simulink library "Swerve_Modules_Controls_Lib"  (R2023a)
settings: Solver=VariableStepAuto  StartTime=0.0  StopTime=10.0  RelTol=1e-3
libraries: Swerve_Drive_lib x4, simulink_extras x4, Rotation2D x4, $bdroot x4, eeGeneralControl x1, slpidlib x1
settings Model: Creator=ander  LastModifiedBy=ander

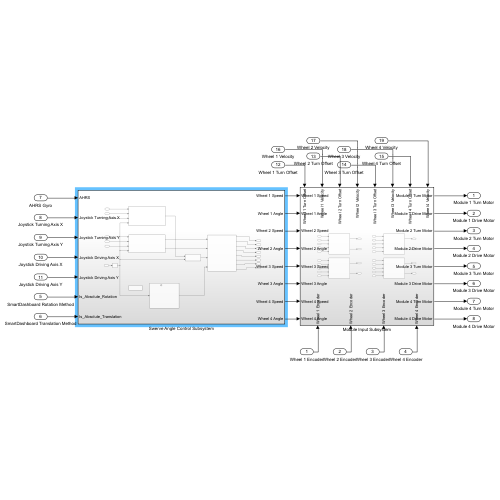
[thumbnail: Simulink's stored preview of the top-level diagram]
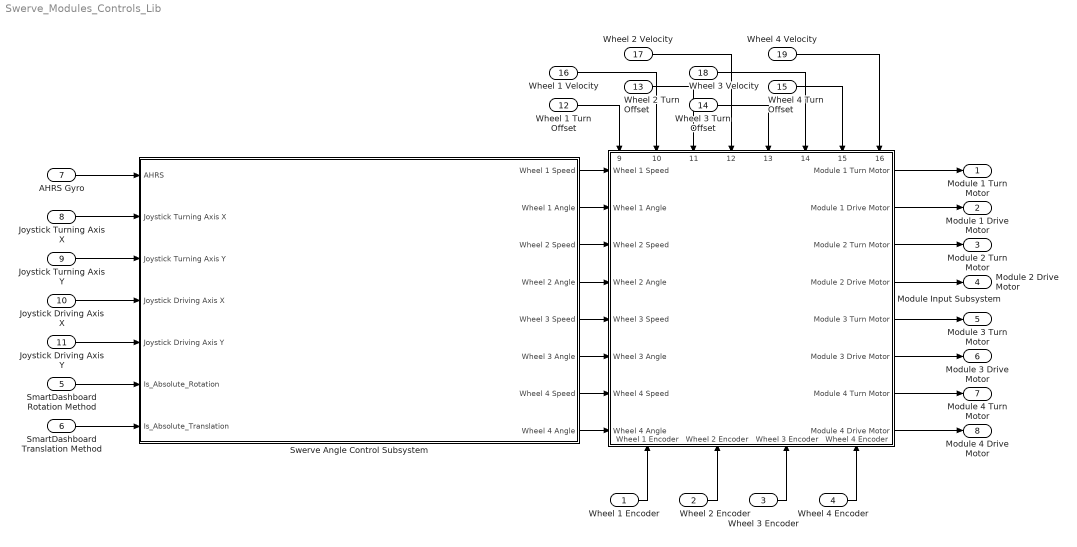
== system Swerve_Modules_Controls_Lib ==
  Wheel 1 Encoder : Inport
  Wheel 2 Encoder : Inport  Port=2
  Wheel 3 Encoder : Inport  Port=3
  Wheel 4 Encoder : Inport  Port=4
  SmartDashboard Rotation Method : Inport  Port=5
  SmartDashboard Translation Method : Inport  Port=6
  AHRS Gyro : Inport  Port=7
  Joystick Turning Axis X : Inport  Port=8
  Joystick Turning Axis Y : Inport  Port=9
  Joystick Driving Axis X : Inport  Port=10
  Joystick Driving Axis Y : Inport  Port=11
  Wheel 1 Turn Offset : Inport  Port=12
  Wheel 2 Turn Offset : Inport  Port=13
  Wheel 3 Turn Offset : Inport  Port=14
  Wheel 4 Turn Offset : Inport  Port=15
  Wheel 1 Velocity : Inport  Port=16
  Wheel 2 Velocity : Inport  Port=17
  Wheel 3 Velocity : Inport  Port=18
  Wheel 4 Velocity : Inport  Port=19
  Module Input Subsystem : Subsystem
      settings: PortSchema="{\"entries\":[{\"content\":{\"sides\":[{\"content\":{\"connectorIds\":[\"In1\",\"In2\",\"In3\",\"In4\",\"In5\",\"In6\",\"In7\",\"In8\"]},\"type\":\"ConnectorPlacement.EquallySpacedRectSide\",\"uuid\":\"43d98aa7-b040-4852-b29d-defb04b38bb2\"},{\"content\":{\"connectorIds\":[\"Out1\",\"Out2\",\"Out3\",\"Out4\",\"Out5\",\"Out6\",\"Out7\",\"Out8\"],\"side\":\"RIGHT\"},\"type\":\"ConnectorPlacement.EquallySpacedRectSide\",\"uuid\":\"cb41fb5c-ab8a-47da-953a-19fc3d1ad3d6\"},{\"content\":{\"connectorIds\":[\"In9\",\"In10\",\"In11\",\"In12\",\"In13\",\"In14\",\"In15\",\"In16\"],\"side\":\"TOP\"},\"type\":\"ConnectorPlacement.EquallySpacedRectSide\",\"uuid\":\"495c5582-c95d-45e8-a83d-3ddc2229b4de\"},{\"content\":{\"connectorIds\":[\"In17\",\"In18\",\"In19\",\"In20\"],\"side\":\"BOTTOM\"},\"type\":\"ConnectorPlacement.EquallySpacedRectSide\",\"uuid\":\"c356cfa6-29bf-4b1b-9842-1083247295af\"}]},\"type\":\"ConnectorPlacement.EquallySpacedConnector\",\"uuid\":\"1f745937-a7fb-445d-9d3d-b08fd0374c25\"}],\"packageUris\":[\"http://schema.mathworks.com/mf0/Connector/R2020b\"],\"version\":\"1.0\"}"
  Swerve Angle Control Subsystem : Subsystem
  Module 1 Turn Motor : Outport
  Module 1 Drive Motor : Outport  Port=2
  Module 2 Turn Motor : Outport  Port=3
  Module 2 Drive Motor : Outport  Port=4
  Module 3 Turn Motor : Outport  Port=5
  Module 3 Drive Motor : Outport  Port=6
  Module 4 Turn Motor : Outport  Port=7
  Module 4 Drive Motor : Outport  Port=8
  wires:
  Swerve Angle Control Subsystem/8(Wheel 4 Angle) -> Module Input Subsystem/8(Wheel 4 Angle)
  Swerve Angle Control Subsystem/7(Wheel 4 Speed) -> Module Input Subsystem/7(Wheel 4 Speed)
  Swerve Angle Control Subsystem/5(Wheel 3 Speed) -> Module Input Subsystem/5(Wheel 3 Speed)
  Swerve Angle Control Subsystem/4(Wheel 2 Angle) -> Module Input Subsystem/4(Wheel 2 Angle)
  Swerve Angle Control Subsystem/3(Wheel 2 Speed) -> Module Input Subsystem/3(Wheel 2 Speed)
  Swerve Angle Control Subsystem/6(Wheel 3 Angle) -> Module Input Subsystem/6(Wheel 3 Angle)
  Swerve Angle Control Subsystem/2(Wheel 1 Angle) -> Module Input Subsystem/2(Wheel 1 Angle)
  Swerve Angle Control Subsystem/1(Wheel 1 Speed) -> Module Input Subsystem/1(Wheel 1 Speed)
  Wheel 1 Encoder/1 -> Module Input Subsystem/17(Wheel 1 Encoder)
  Wheel 2 Encoder/1 -> Module Input Subsystem/18(Wheel 2 Encoder)
  Wheel 3 Encoder/1 -> Module Input Subsystem/19(Wheel 3 Encoder)
  Wheel 4 Encoder/1 -> Module Input Subsystem/20(Wheel 4 Encoder)
  SmartDashboard Rotation Method/1 -> Swerve Angle Control Subsystem/6(Is_Absolute_Rotation)
  SmartDashboard Translation Method/1 -> Swerve Angle Control Subsystem/7(Is_Absolute_Translation)
  AHRS Gyro/1 -> Swerve Angle Control Subsystem/1(AHRS)
  Joystick Turning Axis Y/1 -> Swerve Angle Control Subsystem/3(Joystick Turning Axis Y)
  Joystick Turning Axis X/1 -> Swerve Angle Control Subsystem/2(Joystick Turning Axis X)
  Joystick Driving Axis X/1 -> Swerve Angle Control Subsystem/4(Joystick Driving Axis X)
  Joystick Driving Axis Y/1 -> Swerve Angle Control Subsystem/5(Joystick Driving Axis Y)
  Module Input Subsystem/1(Module 1 Turn Motor) -> Module 1 Turn Motor/1
  Module Input Subsystem/6(Module 3 Drive Motor) -> Module 3 Drive Motor/1
  Module Input Subsystem/5(Module 3 Turn Motor) -> Module 3 Turn Motor/1
  Module Input Subsystem/4(Module 2 Drive Motor) -> Module 2 Drive Motor/1
  Module Input Subsystem/7(Module 4 Turn Motor) -> Module 4 Turn Motor/1
  Module Input Subsystem/8(Module 4 Drive Motor) -> Module 4 Drive Motor/1
  Module Input Subsystem/2(Module 1 Drive Motor) -> Module 1 Drive Motor/1
  Module Input Subsystem/3(Module 2 Turn Motor) -> Module 2 Turn Motor/1
  Wheel 1 Turn Offset/1 -> Module Input Subsystem/9(Wheel 1 Turn Offset)
  Wheel 1 Velocity/1 -> Module Input Subsystem/10(Wheel 1 Velocity)
  Wheel 2 Turn Offset/1 -> Module Input Subsystem/11(Wheel 2 Turn Offset)
  Wheel 2 Velocity/1 -> Module Input Subsystem/12(Wheel 2 Velocity)
  Wheel 3 Turn Offset/1 -> Module Input Subsystem/13(Wheel 3 Turn Offset)
  Wheel 3 Velocity/1 -> Module Input Subsystem/14(Wheel 3 Velocity)
  Wheel 4 Turn Offset/1 -> Module Input Subsystem/15(Wheel 4 Turn Offset)
  Wheel 4 Velocity/1 -> Module Input Subsystem/16(Wheel 4 Velocity)

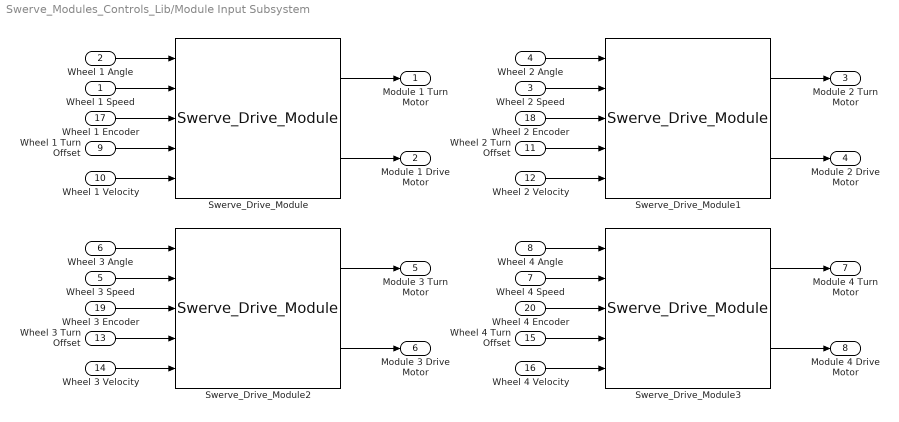
== system Swerve_Modules_Controls_Lib/Module Input Subsystem ==
  Wheel 1 Speed : Inport
  Wheel 1 Angle : Inport  Port=2
  Wheel 2 Speed : Inport  Port=3
  Wheel 2 Angle : Inport  Port=4
  Wheel 3 Speed : Inport  Port=5
  Wheel 3 Angle : Inport  Port=6
  Wheel 4 Speed : Inport  Port=7
  Wheel 4 Angle : Inport  Port=8
  Wheel 1 Turn Offset : Inport  Port=9
  Wheel 1 Velocity : Inport  Port=10
  Wheel 2 Turn Offset : Inport  Port=11
  Wheel 2 Velocity : Inport  Port=12
  Wheel 3 Turn Offset : Inport  Port=13
  Wheel 3 Velocity : Inport  Port=14
  Wheel 4 Turn Offset : Inport  Port=15
  Wheel 4 Velocity : Inport  Port=16
  Wheel 1 Encoder : Inport  Port=17
  Wheel 2 Encoder : Inport  Port=18
  Wheel 3 Encoder : Inport  Port=19
  Wheel 4 Encoder : Inport  Port=20
  Swerve_Drive_Module{,1..3} (4 alike) : Swerve_Drive_lib/Swerve_Drive_Module  SystemSampleTime=-1  VariantActivationTime=update diagram  Latency=0  AutoFrameSizeCalculation=off
  Module 1 Turn Motor : Outport
  Module 1 Drive Motor : Outport  Port=2
  Module 2 Turn Motor : Outport  Port=3
  Module 2 Drive Motor : Outport  Port=4
  Module 3 Turn Motor : Outport  Port=5
  Module 3 Drive Motor : Outport  Port=6
  Module 4 Turn Motor : Outport  Port=7
  Module 4 Drive Motor : Outport  Port=8
  wires:
  Wheel 1 Speed/1 -> Swerve_Drive_Module/2
  Wheel 1 Angle/1 -> Swerve_Drive_Module/1
  Wheel 1 Encoder/1 -> Swerve_Drive_Module/3
  Wheel 2 Encoder/1 -> Swerve_Drive_Module1/3
  Wheel 2 Speed/1 -> Swerve_Drive_Module1/2
  Wheel 2 Angle/1 -> Swerve_Drive_Module1/1
  Wheel 3 Encoder/1 -> Swerve_Drive_Module2/3
  Wheel 3 Speed/1 -> Swerve_Drive_Module2/2
  Wheel 3 Angle/1 -> Swerve_Drive_Module2/1
  Wheel 4 Encoder/1 -> Swerve_Drive_Module3/3
  Wheel 4 Speed/1 -> Swerve_Drive_Module3/2
  Wheel 4 Angle/1 -> Swerve_Drive_Module3/1
  Swerve_Drive_Module/1 -> Module 1 Turn Motor/1
  Swerve_Drive_Module/2 -> Module 1 Drive Motor/1
  Swerve_Drive_Module2/1 -> Module 3 Turn Motor/1
  Swerve_Drive_Module2/2 -> Module 3 Drive Motor/1
  Swerve_Drive_Module1/2 -> Module 2 Drive Motor/1
  Swerve_Drive_Module3/2 -> Module 4 Drive Motor/1
  Swerve_Drive_Module1/1 -> Module 2 Turn Motor/1
  Swerve_Drive_Module3/1 -> Module 4 Turn Motor/1
  Wheel 1 Turn Offset/1 -> Swerve_Drive_Module/4
  Wheel 1 Velocity/1 -> Swerve_Drive_Module/5
  Wheel 2 Turn Offset/1 -> Swerve_Drive_Module1/4
  Wheel 2 Velocity/1 -> Swerve_Drive_Module1/5
  Wheel 3 Turn Offset/1 -> Swerve_Drive_Module2/4
  Wheel 3 Velocity/1 -> Swerve_Drive_Module2/5
  Wheel 4 Turn Offset/1 -> Swerve_Drive_Module3/4
  Wheel 4 Velocity/1 -> Swerve_Drive_Module3/5

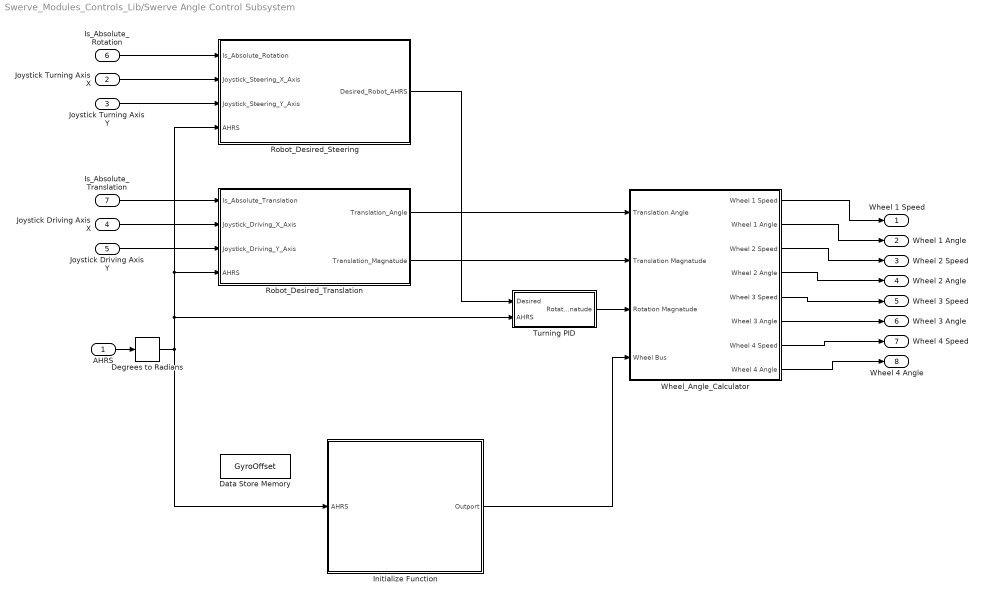
== system Swerve_Modules_Controls_Lib/Swerve Angle Control Subsystem ==
  AHRS : Inport
  Joystick Turning Axis X : Inport  Port=2
  Joystick Turning Axis Y : Inport  Port=3
  Joystick Driving Axis X : Inport  Port=4
  Joystick Driving Axis Y : Inport  Port=5
  Is_Absolute_Rotation : Inport  Port=6  OutDataTypeStr=boolean
  Is_Absolute_Translation : Inport  Port=7  OutDataTypeStr=boolean
  Data Store Memory : DataStoreMemory  DataStoreName=GyroOffset  WriteAfterWriteMsg=warning  ShowAdditionalParam=off  OutDataTypeStr=double
  Degrees to Radians : simulink_extras/Transformations/Degrees to Radians
  Initialize Function : Subsystem  TreatAsAtomicUnit=on
  Robot_Desired_Steering : Subsystem
  Robot_Desired_Translation : Subsystem
  Turning PID : Subsystem
  Wheel_Angle_Calculator : Subsystem
  Wheel 1 Speed : Outport
  Wheel 1 Angle : Outport  Port=2
  Wheel 2 Speed : Outport  Port=3
  Wheel 2 Angle : Outport  Port=4
  Wheel 3 Speed : Outport  Port=5
  Wheel 3 Angle : Outport  Port=6
  Wheel 4 Speed : Outport  Port=7
  Wheel 4 Angle : Outport  Port=8
  wires:
  AHRS/1 -> Degrees to Radians/1
  Degrees to Radians/1 -> Robot_Desired_Translation/4(AHRS), Robot_Desired_Steering/4(AHRS), Turning PID/2(AHRS), Initialize Function/1(AHRS)
  Joystick Driving Axis Y/1 -> Robot_Desired_Translation/3(Joystick_Driving_Y_Axis)
  Joystick Driving Axis X/1 -> Robot_Desired_Translation/2(Joystick_Driving_X_Axis)
  Turning PID/1(Rotation Magnatude) -> Wheel_Angle_Calculator/3(Rotation Magnatude)
  Initialize Function/1(Outport) -> Wheel_Angle_Calculator/4(Wheel Bus)
  Wheel_Angle_Calculator/8(Wheel 4 Angle) -> Wheel 4 Angle/1
  Wheel_Angle_Calculator/7(Wheel 4 Speed) -> Wheel 4 Speed/1
  Wheel_Angle_Calculator/6(Wheel 3 Angle) -> Wheel 3 Angle/1
  Wheel_Angle_Calculator/5(Wheel 3 Speed) -> Wheel 3 Speed/1
  Wheel_Angle_Calculator/4(Wheel 2 Angle) -> Wheel 2 Angle/1
  Wheel_Angle_Calculator/1(Wheel 1 Speed) -> Wheel 1 Speed/1
  Wheel_Angle_Calculator/2(Wheel 1 Angle) -> Wheel 1 Angle/1
  Wheel_Angle_Calculator/3(Wheel 2 Speed) -> Wheel 2 Speed/1
  Robot_Desired_Steering/1(Desired_Robot_AHRS) -> Turning PID/1(Desired)
  Joystick Turning Axis X/1 -> Robot_Desired_Steering/2(Joystick_Steering_X_Axis)
  Joystick Turning Axis Y/1 -> Robot_Desired_Steering/3(Joystick_Steering_Y_Axis)
  Is_Absolute_Rotation/1 -> Robot_Desired_Steering/1(Is_Absolute_Rotation)
  Is_Absolute_Translation/1 -> Robot_Desired_Translation/1(Is_Absolute_Translation)
  Robot_Desired_Translation/1(Translation_Angle) -> Wheel_Angle_Calculator/1(Translation Angle)
  Robot_Desired_Translation/2(Translation_Magnatude) -> Wheel_Angle_Calculator/2(Translation Magnatude)

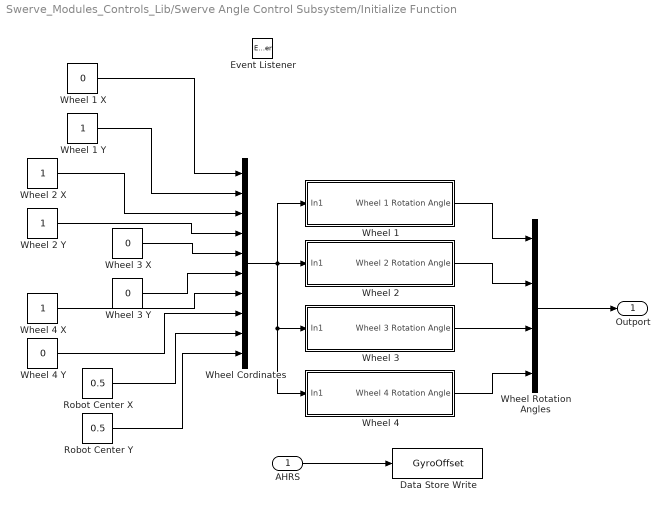
== system Swerve_Modules_Controls_Lib/Swerve Angle Control Subsystem/Initialize Function ==
  AHRS : Inport
  Data Store Write : DataStoreWrite  DataStoreName=GyroOffset  IndexOptions=Index vector (dialog)  Indices=1  OutputSizes=1
  Event Listener : EventListener  DisableCoverage=on  EventName=reset
  Robot Center X : Constant  Value=0.5
  Robot Center Y : Constant  Value=0.5
  Wheel 1 : Subsystem
  Wheel 1 X : Constant  Value=0
  Wheel 1 Y : Constant
  Wheel 2 : Subsystem  AncestorBlock=Swerve_Modules_Controls_Lib/Swerve Motor Control Subsystem/Initialize Function/Wheel 1
      settings: LibrarySourceBlock=Swerve_Modules_Controls_Lib/Swerve Motor Control Subsystem/Initialize Function/Wheel 1
  Wheel 2 X : Constant
  Wheel 2 Y : Constant
  Wheel 3 : Subsystem  AncestorBlock=Swerve_Modules_Controls_Lib/Swerve Motor Control Subsystem/Initialize Function/Wheel 1
      settings: LibrarySourceBlock=Swerve_Modules_Controls_Lib/Swerve Motor Control Subsystem/Initialize Function/Wheel 1
  Wheel 3 X : Constant  Value=0
  Wheel 3 Y : Constant  Value=0
  Wheel 4 : Subsystem  AncestorBlock=Swerve_Modules_Controls_Lib/Swerve Motor Control Subsystem/Initialize Function/Wheel 1
      settings: LibrarySourceBlock=Swerve_Modules_Controls_Lib/Swerve Motor Control Subsystem/Initialize Function/Wheel 1
  Wheel 4 X : Constant
  Wheel 4 Y : Constant  Value=0
  Wheel Cordinates : BusCreator  Inputs=10
  Wheel Rotation Angles : BusCreator  Inputs=4
  Outport : Outport
  wires:
  AHRS/1 -> Data Store Write/1
  Robot Center Y/1 -> Wheel Cordinates/10
  Wheel 4 Y/1 -> Wheel Cordinates/8
  Wheel 4 X/1 -> Wheel Cordinates/7
  Wheel 1 Y/1 -> Wheel Cordinates/2
  Robot Center X/1 -> Wheel Cordinates/9
  Wheel 1 X/1 -> Wheel Cordinates/1
  Wheel 3 Y/1 -> Wheel Cordinates/6
  Wheel 3 X/1 -> Wheel Cordinates/5
  Wheel 2 X/1 -> Wheel Cordinates/3
  Wheel 2 Y/1 -> Wheel Cordinates/4
  Wheel Cordinates/1 -> Wheel 4/1(In1), Wheel 3/1(In1), Wheel 1/1(In1), Wheel 2/1(In1)
  Wheel 1/1(Wheel 1 Rotation Angle) -> Wheel Rotation Angles/1
  Wheel 2/1(Wheel 2 Rotation Angle) -> Wheel Rotation Angles/2
  Wheel 3/1(Wheel 3 Rotation Angle) -> Wheel Rotation Angles/3
  Wheel 4/1(Wheel 4 Rotation Angle) -> Wheel Rotation Angles/4
  Wheel Rotation Angles/1 -> Outport/1

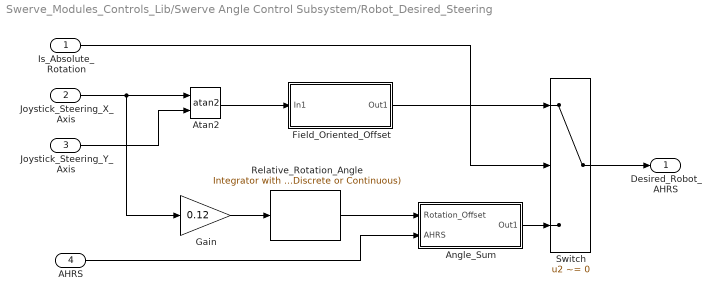
== system Swerve_Modules_Controls_Lib/Swerve Angle Control Subsystem/Robot_Desired_Steering ==
  Is_Absolute_Rotation : Inport
  Joystick_Steering_X_Axis : Inport  Port=2
  Joystick_Steering_Y_Axis : Inport  Port=3
  AHRS : Inport  Port=4
  Angle_Sum : Subsystem
  Atan2 : Trigonometry  Operator=atan2
  Field_Oriented_Offset : Subsystem
  Gain : Gain  Gain=0.12
  Relative_Rotation_Angle : eeGeneralControl/Integrator with Wrapped State (Discrete or Continuous)  LabelModeActiveChoice=Discrete  WrappedStateUpperValue=pi  WrappedStateLowerValue=-pi  x0=0  Ts=-1
      settings: LibrarySourceBlock=|
      | ee_sl_lib/General Control/Integrator with
      | Wrapped State
      | (Discrete or Continuous)
  Switch : Switch  Criteria=u2 ~= 0  SaturateOnIntegerOverflow=off  InputSameDT=off
  Desired_Robot_AHRS : Outport
  wires:
  Relative_Rotation_Angle/1 -> Angle_Sum/1(Rotation_Offset)
  Gain/1 -> Relative_Rotation_Angle/1
  Joystick_Steering_Y_Axis/1 -> Atan2/2
  Field_Oriented_Offset/1(Out1) -> Switch/1
  Angle_Sum/1(Out1) -> Switch/3
  Atan2/1 -> Field_Oriented_Offset/1(In1)
  AHRS/1 -> Angle_Sum/2(AHRS)
  Is_Absolute_Rotation/1 -> Switch/2
  Switch/1 -> Desired_Robot_AHRS/1
  Joystick_Steering_X_Axis/1 -> Gain/1, Atan2/1

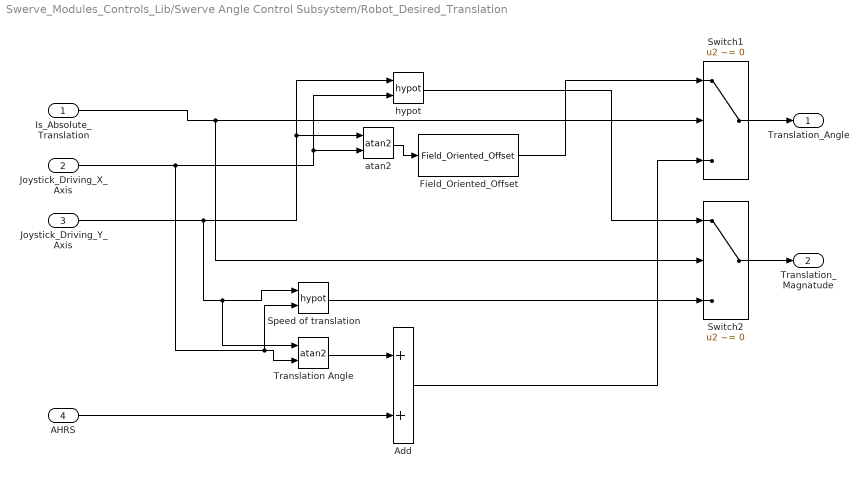
== system Swerve_Modules_Controls_Lib/Swerve Angle Control Subsystem/Robot_Desired_Translation ==
  Is_Absolute_Translation : Inport
  Joystick_Driving_X_Axis : Inport  Port=2
  Joystick_Driving_Y_Axis : Inport  Port=3
  AHRS : Inport  Port=4
  Add : Sum
  Field_Oriented_Offset : $bdroot/Swerve Angle Control Subsystem/Robot_Desired_AHRS_Calc/Field_Oriented_Offset  SystemSampleTime=-1  VariantActivationTime=update diagram  Latency=0  AutoFrameSizeCalculation=off
  Speed of translation : Math  Operator=hypot
  Switch1 : Switch  Criteria=u2 ~= 0  SaturateOnIntegerOverflow=off  InputSameDT=off
  Switch2 : Switch  Criteria=u2 ~= 0  SaturateOnIntegerOverflow=off  InputSameDT=off
  Translation Angle : Trigonometry  Operator=atan2
  atan2 : Trigonometry  Operator=atan2
  hypot : Math  Operator=hypot
  Translation_Angle : Outport
  Translation_Magnatude : Outport  Port=2
  wires:
  Is_Absolute_Translation/1 -> Switch2/2, Switch1/2
  Translation Angle/1 -> Add/1
  Joystick_Driving_Y_Axis/1 -> hypot/1, atan2/1, Speed of translation/1, Translation Angle/1
  Joystick_Driving_X_Axis/1 -> Translation Angle/2, Speed of translation/2, hypot/2, atan2/2
  hypot/1 -> Switch2/1
  atan2/1 -> Field_Oriented_Offset/1
  Switch1/1 -> Translation_Angle/1
  AHRS/1 -> Add/2
  Add/1 -> Switch1/3
  Field_Oriented_Offset/1 -> Switch1/1
  Switch2/1 -> Translation_Magnatude/1
  Speed of translation/1 -> Switch2/3

== system Swerve_Modules_Controls_Lib/Swerve Angle Control Subsystem/Turning PID ==
  note: Needs Tuning
  Desired : Inport
  AHRS : Inport  Port=2
  Minus : Sum  Inputs=+-
  PID Controller : slpidlib/PID Controller  Controller=PID  Form=Parallel  TimeDomain=Continuous-time  UseExternalTs=off  SampleTime=-1  IntegratorMethod=Forward Euler  FilterMethod=Forward Euler  ControllerParametersSource=internal  P=1  I=1  UseKiTs=off  D=0  N=100  UseFilter=on  TunerSelectOption=Transfer Function Based (PID Tuner App)  InitialConditionSource=internal  InitialConditionForIntegrator=0  InitialConditionForFilter=0  DifferentiatorICPrevScaledInput=0  ExternalReset=none  TrackingMode=off  Kt=1  LimitOutput=off  SatLimitsSource=internal  UpperSaturationLimit=inf  LowerSaturationLimit=-inf  LinearizeAsGain=on  AntiWindupMode=none  Kb=1  LimitIntegrator=off  UpperIntegratorSaturationLimit=inf  LowerIntegratorSaturationLimit=-inf  POutMin=[]  POutMax=[]  IOutMin=[]  IOutMax=[]  DOutMin=[]  DOutMax=[]  NOutMin=[]  NOutMax=[]  SumOutMin=[]  SumOutMax=[]  SaturationOutMin=[]  SaturationOutMax=[]  PParamMin=[]  PParamMax=[]  IParamMin=[]  IParamMax=[]  DParamMin=[]  DParamMax=[]  NParamMin=[]  NParamMax=[]  KbParamMin=[]  KbParamMax=[]  KtParamMin=[]  KtParamMax=[]  KbOutMin=[]  KbOutMax=[]  KtOutMin=[]  KtOutMax=[]  IntegratorOutMin=[]  IntegratorOutMax=[]  FilterOutMin=[]  FilterOutMax=[]  SumI1OutMin=[]  SumI1OutMax=[]  SumI2OutMin=[]  SumI2OutMax=[]  SumI3OutMin=[]  SumI3OutMax=[]  SumI4OutMin=[]  SumI4OutMax=[]  SumDOutMin=[]  SumDOutMax=[]  DifferentiatorOutMin=[]  DifferentiatorOutMax=[]  FilterDiffOutCoefMin=[]  FilterDiffOutCoefMax=[]  ReciprocalOutMin=[]  ReciprocalOutMax=[]  SumDenOutMin=[]  SumDenOutMax=[]  SumNumOutMin=[]  SumNumOutMax=[]  DivideOutMin=[]  DivideOutMax=[]  UdiffTsProdOutMin=[]  UdiffTsProdOutMax=[]  NTsProdOutMin=[]  NTsProdOutMax=[]  UintegralTsProdOutMin=[]  UintegralTsProdOutMax=[]  UngainTsProdOutMin=[]  UngainTsProdOutMax=[]  ClampingZeroOutDataTypeStr=Inherit: Inherit via back propagation  ClampingZeroOutMin=[]  ClampingZeroOutMax=[]  FilterDenConstantOutDataTypeStr=Inherit: Inherit via back propagation  FilterDenConstantOutMin=[]  FilterDenConstantOutMax=[]  PCopyOutDataTypeStr=Inherit: Inherit via back propagation  PCopyOutMin=[]  PCopyOutMax=[]  NCopyOutDataTypeStr=Inherit: Inherit via back propagation  NCopyOutMin=[]  NCopyOutMax=[]  IntegratorContinuousStateAttributes=''  IntegratorStateMustResolveToSignalObject=off  IntegratorRTWStateStorageClass=Auto  FilterContinuousStateAttributes=''  FilterStateMustResolveToSignalObject=off  FilterRTWStateStorageClass=Auto  ParallelPVariant=InternalParameters  IdealPVariant=Disabled  IVariant=InternalParameters  DVariant=InternalParameters  IntegratorVariant=Continuous  SatVariant=Disabled  AWVariant=Passthrough  PCopyVariant=Disabled  TRVariant=Disabled  FdbkBlocksVariant=Forward  IdealPFdbkVariant=Disabled  SatFdbkVariant=Disabled  DerivativeFilterVariant=ContFilter  NVariant=InternalParameters  NCopyVariant=Disabled  FilterICVariant=InternalICsFilter  IntegratorICVariant=InternalICs  ExternalResetVariant=Disabled  TRSumVariant=Passthrough  SumFdbkVariant=Disabled  SumVariant=Sum_PID  TsampFilterVariant=InternalTs  TsampNgainVariant=Passthrough  TsampIntegralVariant=Disabled_SignalSpec  ExternalSaturationOutDataTypeStr=Inherit: Same as second input
  Rotation Magnatude : Outport
  wires:
  Desired/1 -> Minus/1
  AHRS/1 -> Minus/2
  Minus/1 -> PID Controller/1
  PID Controller/1 -> Rotation Magnatude/1

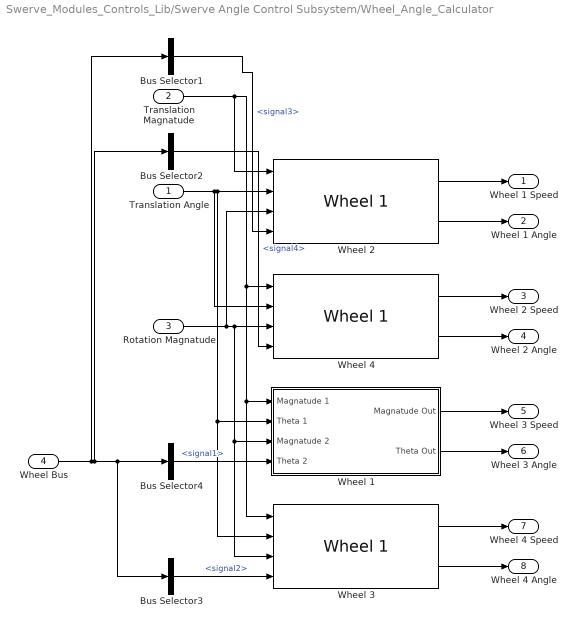
== system Swerve_Modules_Controls_Lib/Swerve Angle Control Subsystem/Wheel_Angle_Calculator ==
  Translation Angle : Inport
  Translation Magnatude : Inport  Port=2
  Rotation Magnatude : Inport  Port=3
  Wheel Bus : Inport  Port=4
  Bus Selector1 : BusSelector  OutputSignals=signal3
  Bus Selector2 : BusSelector  OutputSignals=signal4
  Bus Selector3 : BusSelector  OutputSignals=signal2
  Bus Selector4 : BusSelector  OutputSignals=signal1
  Wheel 1 : Subsystem
  Wheel 2 : $bdroot/Swerve Angle Control Subsystem/Wheel_Angle_Calculator/Wheel 1  SystemSampleTime=-1  VariantActivationTime=update diagram  Latency=0  AutoFrameSizeCalculation=off
  Wheel 3 : $bdroot/Swerve Angle Control Subsystem/Wheel_Angle_Calculator/Wheel 1  SystemSampleTime=-1  VariantActivationTime=update diagram  Latency=0  AutoFrameSizeCalculation=off
  Wheel 4 : $bdroot/Swerve Angle Control Subsystem/Wheel_Angle_Calculator/Wheel 1  SystemSampleTime=-1  VariantActivationTime=update diagram  Latency=0  AutoFrameSizeCalculation=off
  Wheel 1 Speed : Outport
  Wheel 1 Angle : Outport  Port=2
  Wheel 2 Speed : Outport  Port=3
  Wheel 2 Angle : Outport  Port=4
  Wheel 3 Speed : Outport  Port=5
  Wheel 3 Angle : Outport  Port=6
  Wheel 4 Speed : Outport  Port=7
  Wheel 4 Angle : Outport  Port=8
  wires:
  Bus Selector2/1 -> Wheel 4/4  "<signal4>"
  Wheel Bus/1 -> Bus Selector3/1, Bus Selector4/1, Bus Selector2/1, Bus Selector1/1
  Translation Angle/1 -> Wheel 4/2, Wheel 2/2, Wheel 3/2, Wheel 1/2(Theta 1)
  Bus Selector1/1 -> Wheel 2/4  "<signal3>"
  Bus Selector3/1 -> Wheel 3/4  "<signal2>"
  Translation Magnatude/1 -> Wheel 2/1, Wheel 4/1, Wheel 3/1, Wheel 1/1(Magnatude 1)
  Bus Selector4/1 -> Wheel 1/4(Theta 2)  "<signal1>"
  Rotation Magnatude/1 -> Wheel 2/3, Wheel 4/3, Wheel 3/3, Wheel 1/3(Magnatude 2)
  Wheel 3/2 -> Wheel 4 Angle/1
  Wheel 3/1 -> Wheel 4 Speed/1
  Wheel 1/2(Theta Out) -> Wheel 3 Angle/1
  Wheel 1/1(Magnatude Out) -> Wheel 3 Speed/1
  Wheel 4/2 -> Wheel 2 Angle/1
  Wheel 4/1 -> Wheel 2 Speed/1
  Wheel 2/2 -> Wheel 1 Angle/1
  Wheel 2/1 -> Wheel 1 Speed/1

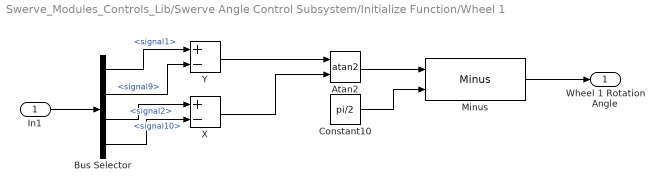
== system Swerve_Modules_Controls_Lib/Swerve Angle Control Subsystem/Initialize Function/Wheel 1 ==
  In1 : Inport
  Atan2 : Trigonometry  Operator=atan2
  Bus Selector : BusSelector  OutputSignals=signal1,signal9,signal2,signal10
  Constant10 : Constant  Value=pi/2
  Minus : Rotation2D/Minus  SystemSampleTime=-1  VariantActivationTime=update diagram  Latency=0  AutoFrameSizeCalculation=off
  X : Sum  Inputs=+-
  Y : Sum  Inputs=+-
  Wheel 1 Rotation Angle : Outport
  wires:
  Atan2/1 -> Minus/1
  Constant10/1 -> Minus/2
  In1/1 -> Bus Selector/1
  Bus Selector/1 -> Y/1  "<signal1>"
  Bus Selector/2 -> Y/2  "<signal9>"
  Bus Selector/3 -> X/1  "<signal2>"
  Bus Selector/4 -> X/2  "<signal10>"
  Y/1 -> Atan2/1
  X/1 -> Atan2/2
  Minus/1 -> Wheel 1 Rotation Angle/1

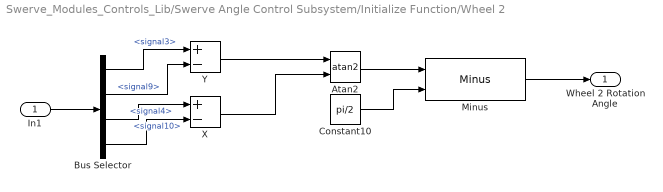
== system Swerve_Modules_Controls_Lib/Swerve Angle Control Subsystem/Initialize Function/Wheel 2 ==
  In1 : Inport
  Atan2 : Trigonometry  Operator=atan2
  Bus Selector : BusSelector  OutputSignals=signal3,signal9,signal4,signal10
  Constant10 : Constant  Value=pi/2
  Minus : Rotation2D/Minus  SystemSampleTime=-1  VariantActivationTime=update diagram  Latency=0  AutoFrameSizeCalculation=off
  X : Sum  Inputs=+-
  Y : Sum  Inputs=+-
  Wheel 2 Rotation Angle : Outport
  wires:
  Atan2/1 -> Minus/1
  Constant10/1 -> Minus/2
  In1/1 -> Bus Selector/1
  Bus Selector/1 -> Y/1  "<signal3>"
  Bus Selector/2 -> Y/2  "<signal9>"
  Bus Selector/3 -> X/1  "<signal4>"
  Bus Selector/4 -> X/2  "<signal10>"
  Y/1 -> Atan2/1
  X/1 -> Atan2/2
  Minus/1 -> Wheel 2 Rotation Angle/1

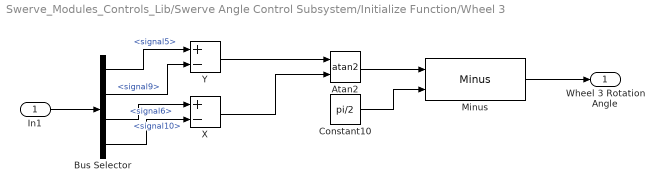
== system Swerve_Modules_Controls_Lib/Swerve Angle Control Subsystem/Initialize Function/Wheel 3 ==
  In1 : Inport
  Atan2 : Trigonometry  Operator=atan2
  Bus Selector : BusSelector  OutputSignals=signal5,signal9,signal6,signal10
  Constant10 : Constant  Value=pi/2
  Minus : Rotation2D/Minus  SystemSampleTime=-1  VariantActivationTime=update diagram  Latency=0  AutoFrameSizeCalculation=off
  X : Sum  Inputs=+-
  Y : Sum  Inputs=+-
  Wheel 3 Rotation Angle : Outport
  wires:
  Atan2/1 -> Minus/1
  Constant10/1 -> Minus/2
  In1/1 -> Bus Selector/1
  Bus Selector/1 -> Y/1  "<signal5>"
  Bus Selector/2 -> Y/2  "<signal9>"
  Bus Selector/3 -> X/1  "<signal6>"
  Bus Selector/4 -> X/2  "<signal10>"
  Y/1 -> Atan2/1
  X/1 -> Atan2/2
  Minus/1 -> Wheel 3 Rotation Angle/1

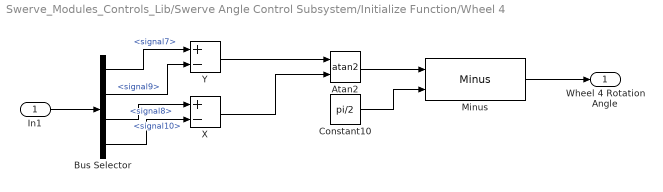
== system Swerve_Modules_Controls_Lib/Swerve Angle Control Subsystem/Initialize Function/Wheel 4 ==
  In1 : Inport
  Atan2 : Trigonometry  Operator=atan2
  Bus Selector : BusSelector  OutputSignals=signal7,signal9,signal8,signal10
  Constant10 : Constant  Value=pi/2
  Minus : Rotation2D/Minus  SystemSampleTime=-1  VariantActivationTime=update diagram  Latency=0  AutoFrameSizeCalculation=off
  X : Sum  Inputs=+-
  Y : Sum  Inputs=+-
  Wheel 4 Rotation Angle : Outport
  wires:
  Atan2/1 -> Minus/1
  Constant10/1 -> Minus/2
  In1/1 -> Bus Selector/1
  Bus Selector/1 -> Y/1  "<signal7>"
  Bus Selector/2 -> Y/2  "<signal9>"
  Bus Selector/3 -> X/1  "<signal8>"
  Bus Selector/4 -> X/2  "<signal10>"
  Y/1 -> Atan2/1
  X/1 -> Atan2/2
  Minus/1 -> Wheel 4 Rotation Angle/1

== system Swerve_Modules_Controls_Lib/Swerve Angle Control Subsystem/Robot_Desired_Steering/Angle_Sum ==
  Rotation_Offset : Inport
  AHRS : Inport  Port=2
  Integrator : Integrator  InitialConditionSource=external  WrapState=on
  Out1 : Outport
  wires:
  Rotation_Offset/1 -> Integrator/1
  Integrator/1 -> Out1/1
  AHRS/1 -> Integrator/2

== system Swerve_Modules_Controls_Lib/Swerve Angle Control Subsystem/Robot_Desired_Steering/Field_Oriented_Offset ==
  In1 : Inport
  Data Store Read : DataStoreRead  DataStoreName=GyroOffset  IndexOptions=Index vector (dialog)  Indices=1  OutputSizes=1
  Integrator : Integrator  InitialConditionSource=external  WrapState=on
  Out1 : Outport
  wires:
  In1/1 -> Integrator/2
  Integrator/1 -> Out1/1
  Data Store Read/1 -> Integrator/1

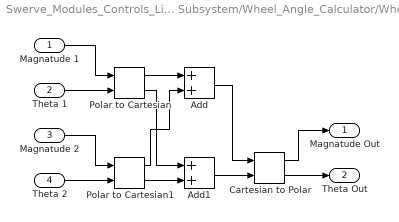
== system Swerve_Modules_Controls_Lib/Swerve Angle Control Subsystem/Wheel_Angle_Calculator/Wheel 1 ==
  Magnatude 1 : Inport
  Theta 1 : Inport  Port=2
  Magnatude 2 : Inport  Port=3
  Theta 2 : Inport  Port=4
  Add : Sum
  Add1 : Sum
  Cartesian to Polar : simulink_extras/Transformations/Cartesian to Polar
  Polar to Cartesian : simulink_extras/Transformations/Polar to Cartesian
  Polar to Cartesian1 : simulink_extras/Transformations/Polar to Cartesian
  Magnatude Out : Outport
  Theta Out : Outport  Port=2
  wires:
  Magnatude 1/1 -> Polar to Cartesian/1
  Polar to Cartesian1/1 -> Add/2
  Polar to Cartesian/2 -> Add1/1
  Magnatude 2/1 -> Polar to Cartesian1/1
  Theta 1/1 -> Polar to Cartesian/2
  Polar to Cartesian/1 -> Add/1
  Polar to Cartesian1/2 -> Add1/2
  Theta 2/1 -> Polar to Cartesian1/2
  Add/1 -> Cartesian to Polar/1
  Add1/1 -> Cartesian to Polar/2
  Cartesian to Polar/1 -> Magnatude Out/1
  Cartesian to Polar/2 -> Theta Out/1
